simulink model "lab_two_task_two"  (R2018b)
settings: Solver=FixedStepDiscrete  StartTime=0.0  StopTime=10.0  RelTol=1e-3
settings Model: Creator=Romario  LastModifiedBy=Romario
settings OptimizationCC: DefaultParameterBehavior=Inlined  EnhancedBackFolding=on  PassReuseOutputArgsAs=Individual arguments  OptimizeBlockOrder=speed  DifferentSizesBufferReuse=on  OptimizationCustomize=off
settings DebuggingCC: UnderspecifiedInitializationDetection=Classic  MergeDetectMultiDrivingBlocksExec=none  ParameterTunabilityLossMsg=error
settings ModelReferenceCC: PropagateSignalLabelsOutOfModel=off
settings SFSimCC: MATLABDynamicMemAlloc=off
settings RTWCC: SystemTargetFile=ert.tlc  GenCodeOnly=on  TemplateMakefile=ert_default_tmf  GenerateReport=on  IncludeHyperlinkInReport=on  LaunchReport=on  GenerateTraceInfo=on  GenerateTraceReport=on  GenerateTraceReportSl=on  GenerateTraceReportSf=on  GenerateTraceReportEml=on
settings CodeAppCC: ForceParamTrailComments=on  IgnoreCustomStorageClasses=off  OperatorAnnotations=on  SimulinkDataObjDesc=on  SFDataObjDesc=on  InsertBlockDesc=on
settings ERTTargetCC: TargetLangStandard=C99 (ISO)  GenerateSampleERTMain=on  InlinedParameterPlacement=NonHierarchical  ERTCustomFileTemplate=example_file_process.tlc

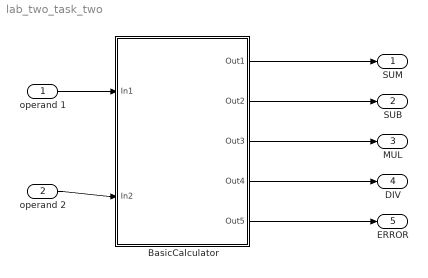
== system lab_two_task_two ==
  "operand 1 " : Inport
  operand 2 : Inport  Port=2
  BasicCalculator : Subsystem  TreatAsAtomicUnit=on
      settings: MinAlgLoopOccurrences=on  RTWFcnNameOpts=Use subsystem name
  SUM : Outport
  SUB : Outport  Port=2
  MUL : Outport  Port=3
  DIV : Outport  Port=4
  "ERROR " : Outport  Port=5  SignalName=ERROR
  wires:
  "operand 1 "/1 -> BasicCalculator/1(In1)
  operand 2/1 -> BasicCalculator/2(In2)
  BasicCalculator/1(Out1) -> SUM/1
  BasicCalculator/2(Out2) -> SUB/1
  BasicCalculator/3(Out3) -> MUL/1
  BasicCalculator/4(Out4) -> DIV/1
  BasicCalculator/5(Out5) -> "ERROR "/1

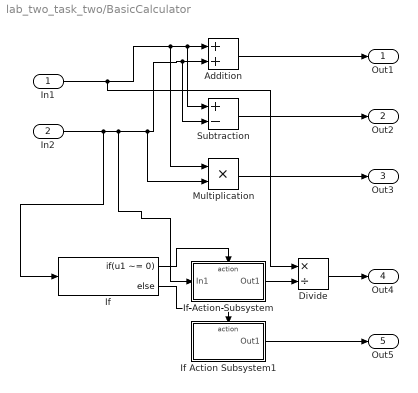
== system lab_two_task_two/BasicCalculator ==
  In1 : Inport
  In2 : Inport  Port=2
  Addition : Sum
  Divide : Product  Inputs=*/
  If : If  IfExpression=u1 ~= 0
  If Action Subsystem : Subsystem  TreatAsAtomicUnit=on
  If Action Subsystem1 : Subsystem  TreatAsAtomicUnit=on
  "Multiplication " : Product
  "Subtraction " : Sum  Inputs=+-
  Out1 : Outport
  Out2 : Outport  Port=2
  Out3 : Outport  Port=3
  Out4 : Outport  Port=4
  Out5 : Outport  Port=5
  wires:
  "Subtraction "/1 -> Out2/1
  In1/1 -> Divide/1, "Multiplication "/1, "Subtraction "/1, Addition/1
  In2/1 -> If/1, If Action Subsystem/1(In1), "Multiplication "/2, "Subtraction "/2, Addition/2
  If/2 -> If Action Subsystem1/Action
  "Multiplication "/1 -> Out3/1
  If Action Subsystem/1(Out1) -> Divide/2
  If/1 -> If Action Subsystem/Action
  Divide/1 -> Out4/1
  Addition/1 -> Out1/1
  If Action Subsystem1/1(Out1) -> Out5/1

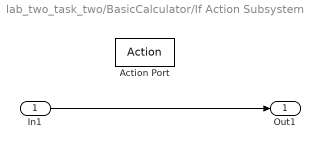
== system lab_two_task_two/BasicCalculator/If Action Subsystem ==
  In1 : Inport
  Action Port : ActionPort  ActionType=then
  Out1 : Outport
  wires:
  In1/1 -> Out1/1

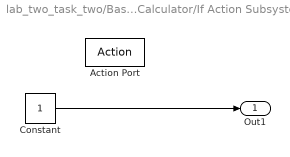
== system lab_two_task_two/BasicCalculator/If Action Subsystem1 ==
  Action Port : ActionPort  ActionType=else
  Constant : Constant
  Out1 : Outport
  wires:
  Constant/1 -> Out1/1
